simulink model "lab5_1"  (R2020b)
settings: Solver=ode23s  StartTime=0.0  StopTime=0.1  RelTol=1e-5
libraries: powerlib x11, simulink x3
settings Model: Creator=Le tueur  LastModifiedBy=Le tueur

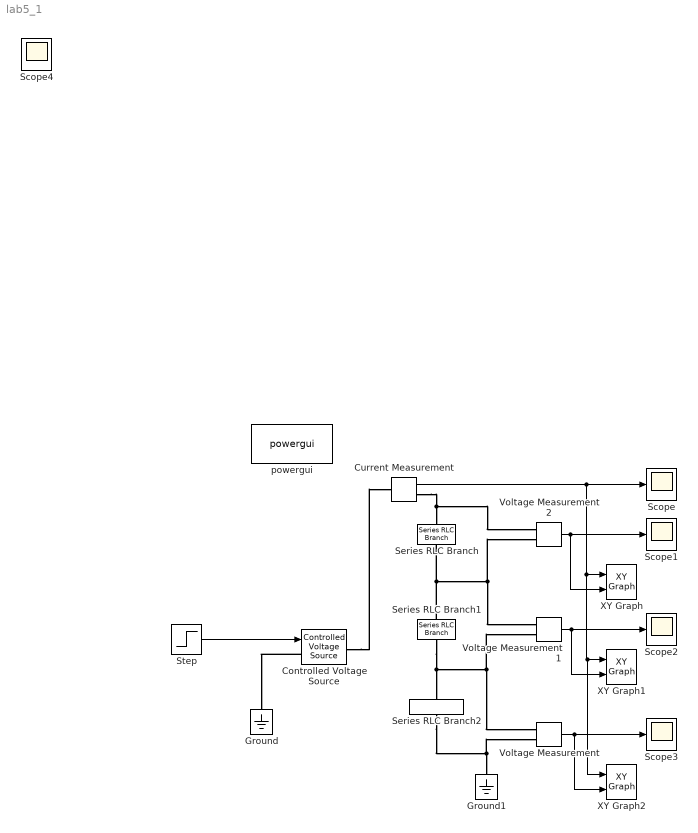
== system lab5_1 ==
  Controlled Voltage Source : powerlib/Electrical Sources/Controlled Voltage Source  Initialize=on  Source_Type=AC  Amplitude=0  Phase=0  Frequency=0  Measurements=None
  Current Measurement : powerlib/Measurements/Current Measurement  PhasorSimulation=off  OutputType=Complex  PSBequivalent=0
  Ground : powerlib/Elements/Ground  LConnTagsString=a
  Ground1 : powerlib/Elements/Ground  LConnTagsString=a
  Scope{,1..4} (5 alike) : Scope
  Series RLC Branch : powerlib/Elements/Series RLC Branch  LConnTagsString=__new0  RConnTagsString=__new0  BranchType=R  Resistance=0.9  Inductance=0  SetiL0=off  InitialCurrent=0  Capacitance=0  Setx0=off  InitialVoltage=0  Measurements=None
  Series RLC Branch1 : powerlib/Elements/Series RLC Branch  LConnTagsString=__new0  RConnTagsString=__new0  BranchType=L  Resistance=1  Inductance=1e-2  SetiL0=off  InitialCurrent=0  Capacitance=1e-6  Setx0=off  InitialVoltage=0  Measurements=None
  Series RLC Branch2 : powerlib/Elements/Series RLC Branch  LConnTagsString=__new0  RConnTagsString=__new0  BranchType=C  Resistance=1  Inductance=1e-3  SetiL0=off  InitialCurrent=0  Capacitance=1e-3  Setx0=off  InitialVoltage=0  Measurements=None
  Step : Step  Time=0.01  After=400  SampleTime=0
  Voltage Measurement : powerlib/Measurements/Voltage Measurement  PhasorSimulation=off  OutputType=Complex  PSBequivalent=0
  Voltage Measurement1 : powerlib/Measurements/Voltage Measurement  PhasorSimulation=off  OutputType=Complex  PSBequivalent=0
  Voltage Measurement2 : powerlib/Measurements/Voltage Measurement  PhasorSimulation=off  OutputType=Complex  PSBequivalent=0
  XY Graph : simulink/Sinks/XY Graph  xmin=-100  xmax=150  ymin=-200  ymax=200  st=-1
  XY Graph1 : simulink/Sinks/XY Graph  xmin=-150  xmax=150  ymin=-400  ymax=500  st=-1
  XY Graph2 : simulink/Sinks/XY Graph  xmin=-150  xmax=150  ymin=-200  ymax=800  st=-1
  powergui : powerlib/powergui  Priority=1  SimulationMode=Continuous  SampleTime=50e-6  frequency=60  Iterations=50  frequencyindice=0  Pbase=100e6  ErrMax=1e-4  UnitsV=kV  UnitsW=MW  buscounter=0  FunctionMessages=off  echomessages=off  EnableUseOfTLC=off  CurrentSourceSwitches=off  DisableSnubberDevices=off  DisableRonSwitches=off  DisableVfSwitches=off  DisplayEquations=off  AutomaticDiscreteSolvers=off  SolverType=Tustin/Backward Euler (TBE)  Interpol=off  ExternalGateDelay=off  methode=off  Ts=100  x0status=blocks  SPID=on  SwTol=0  HookPort=off  NonlinearTolerance=1e-4  nMaxIteration=100  ContinueOnMaxIteration=off  RestoreLinks=warning  ResistiveCurrentMeasurement=off  Frange=[0:2:500]  Ylog=off  Xlog=on  ShowGrid=off  save=off  variable=ZData  structure=0  ZoomFFT=off  StartTime=0.0  cycles=1  DisplayStyle=1  fundamental=60  FreqAxis=off  MaxFrequency=1000  frequencyindicesteady=1  RmsSteady=1  display=off
  wires:
  Current Measurement/1 -> XY Graph/1, XY Graph2/1, XY Graph1/1, Scope/1
  Voltage Measurement2/1 -> XY Graph/2, Scope1/1
  Voltage Measurement1/1 -> XY Graph1/2, Scope2/1
  Voltage Measurement/1 -> XY Graph2/2, Scope3/1
  Step/1 -> Controlled Voltage Source/1
  connections:
  Current Measurement/RConn1 -- Voltage Measurement2/LConn1 -- Series RLC Branch/LConn1
  Series RLC Branch1/LConn1 -- Voltage Measurement1/LConn1 -- Voltage Measurement2/LConn2 -- Series RLC Branch/RConn1
  Series RLC Branch1/RConn1 -- Voltage Measurement1/LConn2 -- Voltage Measurement/LConn1 -- Series RLC Branch2/RConn1
  Series RLC Branch2/LConn1 -- Voltage Measurement/LConn2 -- Ground1/LConn1
  Controlled Voltage Source/RConn1 -- Current Measurement/LConn1
  Controlled Voltage Source/LConn1 -- Ground/LConn1
